simulink model "lab3_2"  (R2023b)
settings: Solver=VariableStepAuto  StartTime=0.0  StopTime=1  MaxStep=0.1  RelTol=1e-3
settings Model: Creator=user  LastModifiedBy=Admin

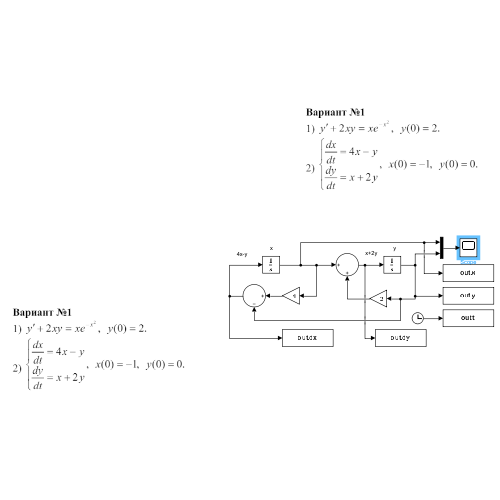
[thumbnail: Simulink's stored preview of the top-level diagram]
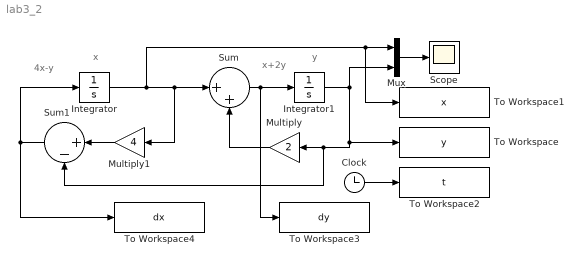
== system lab3_2 ==
  note: x+2y
  note: 4x-y
  note: x
  note: y
  Clock : Clock
  Integrator : Integrator  InitialCondition=-1
  Integrator1 : Integrator
  Multiply : Gain  Gain=2
  Multiply1 : Gain  Gain=4
  Mux : Mux  Inputs=2
  Scope : Scope
  Sum : Sum  Inputs=|++
  Sum1 : Sum  Inputs=|+-
  To Workspace : ToWorkspace  VariableName=y  SampleTime=-1
  To Workspace1 : ToWorkspace  VariableName=x  SampleTime=-1
  To Workspace2 : ToWorkspace  VariableName=t  SampleTime=-1
  To Workspace3 : ToWorkspace  VariableName=dy  SampleTime=-1
  To Workspace4 : ToWorkspace  VariableName=dx  SampleTime=-1
  wires:
  Mux/1 -> Scope/1
  Integrator1/1 -> To Workspace/1, Sum1/2, Multiply/1, Mux/2
  Integrator/1 -> Multiply1/1, Sum/1, To Workspace1/1, Mux/1
  Multiply/1 -> Sum/2
  Sum/1 -> To Workspace3/1, Integrator1/1
  Multiply1/1 -> Sum1/1
  Sum1/1 -> To Workspace4/1, Integrator/1
  Clock/1 -> To Workspace2/1
